simulink library "body_chassis_vert"  (R2018b)
settings: Solver=ode45  StartTime=0.0  StopTime=10.0  RelTol=1e-3  EnableMultiTasking=on
undefined symbols (not defined in the file): DiscIntNeverNeededParam, par_VEH, phi0, psip0, stepsize, v0
libraries: $bdroot x4
(part 2 of 2)

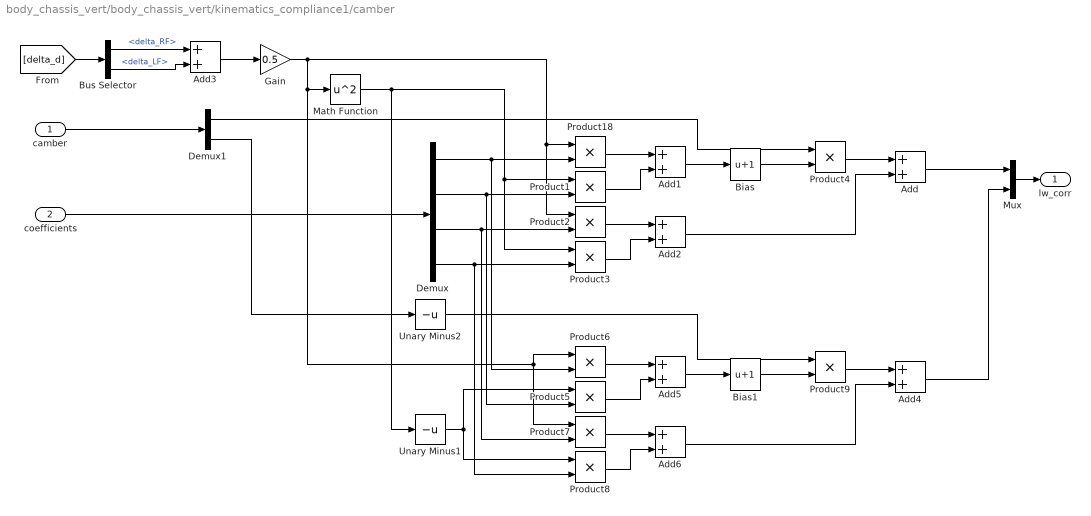
== system body_chassis_vert/body_chassis_vert/kinematics_compliance1/camber ==
  "camber " : Inport
  coefficients : Inport  Port=2
  Add{,1..6} (7 alike) : Sum
  Bias : Bias  Bias=1
  Bias1 : Bias  Bias=1
  Bus Selector : BusSelector  OutputSignals=delta_RF,delta_LF
  Demux : Demux
  Demux1 : Demux  Outputs=2
  Gain : Gain  Gain=0.5
  Math Function : Math  Operator=square  SaturateOnIntegerOverflow=on
  Mux : Mux  Inputs=2
  Product{1..9,18} (10 alike) : Product  RndMeth=Zero
  Unary Minus1 : UnaryMinus
  Unary Minus2 : UnaryMinus
  lw_corr : Outport
  wires:
  Unary Minus2/1 -> Product9/1
  Add3/1 -> Gain/1
  Bus Selector/2 -> Add3/2  "<delta_LF>"
  Bus Selector/1 -> Add3/1  "<delta_RF>"
  [delta_d] -> Bus Selector/1
  "camber "/1 -> Demux1/1
  Add/1 -> Mux/1
  coefficients/1 -> Demux/1
  Demux/1 -> Product6/2, Product18/2
  Demux/2 -> Product5/2, Product1/2
  Math Function/1 -> Unary Minus1/1, Product3/1, Product1/1
  Demux/3 -> Product7/2, Product2/2
  Demux/4 -> Product8/2, Product3/2
  Product18/1 -> Add1/1
  Product1/1 -> Add1/2
  Add1/1 -> Bias/1
  Product2/1 -> Add2/1
  Product3/1 -> Add2/2
  Add2/1 -> Add/2
  Bias/1 -> Product4/2
  Product4/1 -> Add/1
  Demux1/1 -> Product4/1
  Add4/1 -> Mux/2
  Product5/1 -> Add5/2
  Add5/1 -> Bias1/1
  Product7/1 -> Add6/1
  Product8/1 -> Add6/2
  Add6/1 -> Add4/2
  Bias1/1 -> Product9/2
  Product9/1 -> Add4/1
  Gain/1 -> Math Function/1, Product6/1, Product7/1, Product2/1, Product18/1
  Unary Minus1/1 -> Product5/1, Product8/1
  Product6/1 -> Add5/1
  Demux1/2 -> Unary Minus2/1
  Mux/1 -> lw_corr/1

== system body_chassis_vert/body_chassis_vert/kinematics_compliance1/toe ==
  "toe " : Inport
  coefficients : Inport  Port=2
  Add{,1..6} (7 alike) : Sum
  Bias : Bias  Bias=1
  Bias1 : Bias  Bias=1
  Bus Selector : BusSelector  OutputSignals=delta_RF,delta_LF
  Demux : Demux
  Demux1 : Demux  Outputs=2
  Gain : Gain  Gain=0.5
  Math Function : Math  Operator=square  SaturateOnIntegerOverflow=on
  Mux : Mux  Inputs=2
  Product{1..9,18} (10 alike) : Product  RndMeth=Zero
  Unary Minus : UnaryMinus
  Unary Minus2 : UnaryMinus
  lw_corr : Outport
  wires:
  Unary Minus2/1 -> Product9/1
  Mux/1 -> lw_corr/1
  Demux1/2 -> Unary Minus2/1
  Product6/1 -> Add5/1
  Math Function/1 -> Product1/1, Product3/1, Product5/1, Product8/1
  Unary Minus/1 -> Product7/1, Product6/1
  Product9/1 -> Add4/1
  Bias1/1 -> Product9/2
  Add6/1 -> Add4/2
  Product8/1 -> Add6/2
  Product7/1 -> Add6/1
  Add5/1 -> Bias1/1
  Product5/1 -> Add5/2
  Add4/1 -> Mux/2
  Demux1/1 -> Product4/1
  Product4/1 -> Add/1
  Bias/1 -> Product4/2
  Add2/1 -> Add/2
  Product3/1 -> Add2/2
  Product2/1 -> Add2/1
  Add1/1 -> Bias/1
  Product1/1 -> Add1/2
  Product18/1 -> Add1/1
  Demux/4 -> Product3/2, Product8/2
  Demux/3 -> Product2/2, Product7/2
  Demux/2 -> Product1/2, Product5/2
  Gain/1 -> Product18/1, Product2/1, Math Function/1, Unary Minus/1
  Demux/1 -> Product18/2, Product6/2
  coefficients/1 -> Demux/1
  Add/1 -> Mux/1
  "toe "/1 -> Demux1/1
  [delta_d] -> Bus Selector/1
  Bus Selector/1 -> Add3/1  "<delta_RF>"
  Bus Selector/2 -> Add3/2  "<delta_LF>"
  Add3/1 -> Gain/1

== system body_chassis_vert/body_chassis_vert/roll/phi ==
  phi : Inport
  LF : Inport  Port=2
  RF : Inport  Port=3
  RR : Inport  Port=4
  LR : Inport  Port=5
  Product{5..8} (4 alike) : Product  RndMeth=Zero
  Trigonometric Function : Trigonometry
  Unary Minus1 : UnaryMinus
  RF_out : Outport
  LF_out : Outport  Port=2
  RR_out : Outport  Port=3
  LR_out : Outport  Port=4
  wires:
  Product8/1 -> LR_out/1  "z_roll_LR"
  Product7/1 -> RR_out/1  "z_roll_RR"
  Product6/1 -> LF_out/1  "z_roll_LF"
  Product5/1 -> RF_out/1  "z_roll_RF"
  LR/1 -> Product8/2
  RR/1 -> Product7/2
  LF/1 -> Product6/2
  RF/1 -> Product5/2
  phi/1 -> Trigonometric Function/1
  Trigonometric Function/1 -> Product8/1, Product6/1, Unary Minus1/1
  Unary Minus1/1 -> Product5/1, Product7/1

== system body_chassis_vert/body_chassis_vert/suspension/arb ==
  note: Fz_arb_RF is refered to wheel
  z_roll : Inport
  z_wheel_vert : Inport  Port=2
  Bus Creator : BusCreator  Inputs=4
  Front : Subsystem
  Front1 : Subsystem
  F_arb : Outport
  wires:
  [carbR] -> Front1/3(carb)
  Front/2(Fz_arb_L) -> Bus Creator/2  "Fz_arb_LF"
  z_wheel_vert/1 -> Front1/2(z_wheel_vert), Front/2(z_wheel_vert)
  z_roll/1 -> Front1/1(z_roll), Front/1(z_roll)
  Front1/2(Fz_arb_L) -> Bus Creator/4  "Fz_arb_LR"
  Front1/1(Fz_arb_R) -> Bus Creator/3  "Fz_arb_RR"
  Front/1(Fz_arb_R) -> Bus Creator/1  "Fz_arb_RF"
  Bus Creator/1 -> F_arb/1
  [carbF] -> Front/3(carb)

== system body_chassis_vert/body_chassis_vert/suspension/damper ==
  note: Fz_damper is refered to wheel
  z_roll : Inport
  z_pitch : Inport  Port=2
  z_body_vert : Inport  Port=3
  z_wheel_vert : Inport  Port=4
  Bus Creator : BusCreator  Inputs=4
  Bus Creator1 : BusCreator  Inputs=4
  Bus Selector : BusSelector  OutputSignals=z_roll_RF.z_roll_RFp,z_roll_LF.z_roll_LFp,z_roll_RR.z_roll_RRp,z_roll_LR.z_roll_LRp
  Bus Selector1 : BusSelector  OutputSignals=z_pitch_RF.z_pitch_RFp,z_pitch_LF.z_pitch_LFp,z_pitch_RR.z_pitch_RRp,z_pitch_LR.z_pitch_LRp
  Bus Selector2 : BusSelector  OutputSignals=z_vertp
  Bus Selector3 : BusSelector  OutputSignals=zwheel_RF.zwheelp,zwheel_LF.zwheelp,zwheel_RR.zwheelp,zwheel_LR.zwheelp
  LF : Subsystem
  LR : Subsystem
  RF : Subsystem
  RR : Subsystem
  F_damper : Outport
  P_damper : Outport  Port=2
  wires:
  Bus Selector3/3 -> RR/4(z_wheel_vertp)  "<zwheelp>"
  Bus Selector3/2 -> LF/4(z_wheel_vertp)  "<zwheelp>"
  Bus Selector3/1 -> RF/4(z_wheel_vertp)  "<zwheelp>"
  Bus Selector/4 -> LR/1(z_rollp)  "<z_roll_LRp>"
  Bus Selector/3 -> RR/1(z_rollp)  "<z_roll_RRp>"
  Bus Selector/2 -> LF/1(z_rollp)  "<z_roll_LFp>"
  Bus Selector/1 -> RF/1(z_rollp)  "<z_roll_RFp>"
  Bus Selector1/1 -> RF/2(z_pitchp)  "<z_pitch_RFp>"
  Bus Selector1/2 -> LF/2(z_pitchp)  "<z_pitch_LFp>"
  Bus Selector1/3 -> RR/2(z_pitchp)  "<z_pitch_RRp>"
  Bus Selector1/4 -> LR/2(z_pitchp)  "<z_pitch_LRp>"
  Bus Selector3/4 -> LR/4(z_wheel_vertp)  "<zwheelp>"
  Bus Selector2/1 -> LR/3(z_vertp), RR/3(z_vertp), LF/3(z_vertp), RF/3(z_vertp)  "<z_vertp>"
  z_body_vert/1 -> Bus Selector2/1
  RF/1(Fz_damper) -> Bus Creator/1  "Fz_damper_RF"
  LF/1(Fz_damper) -> Bus Creator/2  "Fz_damper_LF"
  RR/1(Fz_damper) -> Bus Creator/3  "Fz_damper_RR"
  LR/1(Fz_damper) -> Bus Creator/4  "Fz_damper_LR"
  z_roll/1 -> Bus Selector/1
  z_pitch/1 -> Bus Selector1/1
  Bus Creator/1 -> F_damper/1
  z_wheel_vert/1 -> Bus Selector3/1
  Bus Creator1/1 -> P_damper/1
  RF/2(P_damper) -> Bus Creator1/1  "P_damper_RF"
  LF/2(P_damper) -> Bus Creator1/2  "P_damper_LF"
  RR/2(P_damper) -> Bus Creator1/3  "P_damper_RR"
  LR/2(P_damper) -> Bus Creator1/4  "P_damper_LR"

== system body_chassis_vert/body_chassis_vert/suspension/spring ==
  note: Fz_spring is refered to wheel
  z_roll : Inport
  z_pitch : Inport  Port=2
  z_vert : Inport  Port=3
  z_wheel_vert : Inport  Port=4
  Bus Creator : BusCreator  Inputs=4
  Bus Creator1 : BusCreator  Inputs=4
  Bus Selector : BusSelector  OutputSignals=z_roll_RF.z_roll_RF,z_roll_LF.z_roll_LF,z_roll_RR.z_roll_RR,z_roll_LR.z_roll_LR
  Bus Selector1 : BusSelector  OutputSignals=z_pitch_RF.z_pitch_RF,z_pitch_LF.z_pitch_LF,z_pitch_RR.z_pitch_RR,z_pitch_LR.z_pitch_LR
  Bus Selector2 : BusSelector  OutputSignals=z_vert
  Bus Selector3 : BusSelector  OutputSignals=zwheel_RF.zwheel,zwheel_LF.zwheel,zwheel_RR.zwheel,zwheel_LR.zwheel
  LF : $bdroot/body_chassis_vert/suspension/spring/RF  SystemSampleTime=-1
  LR : $bdroot/body_chassis_vert/suspension/spring/RR  SystemSampleTime=-1
  RF : Subsystem
  RR : Subsystem
  Fz_spring : Outport
  z_wheel : Outport  Port=2
  wires:
  z_pitch/1 -> Bus Selector1/1
  LR/2 -> Bus Creator1/4  "z_wheel_LR"
  RR/2(z_wheel) -> Bus Creator1/3  "z_wheel_RR"
  LF/2 -> Bus Creator1/2  "z_wheel_LF"
  RF/2(z_wheel) -> Bus Creator1/1  "z_wheel_RF"
  Bus Creator1/1 -> z_wheel/1
  Bus Selector2/1 -> RF/3(z_vert), LF/3, LR/2, RR/3(z_vert)  "<z_vert>"
  Bus Selector3/4 -> LR/4  "<zwheel>"
  Bus Selector3/3 -> RR/4(z_wheel_vert)  "<zwheel>"
  z_wheel_vert/1 -> Bus Selector3/1
  Bus Selector3/1 -> RF/4(z_wheel_vert)  "<zwheel>"
  z_vert/1 -> Bus Selector2/1
  Bus Creator/1 -> Fz_spring/1
  Bus Selector1/4 -> LR/3  "<z_pitch_LR>"
  Bus Selector1/3 -> RR/2(z_pitch)  "<z_pitch_RR>"
  Bus Selector1/2 -> LF/2  "<z_pitch_LF>"
  Bus Selector1/1 -> RF/2(z_pitch)  "<z_pitch_RF>"
  Bus Selector/4 -> LR/1  "<z_roll_LR>"
  Bus Selector/3 -> RR/1(z_roll)  "<z_roll_RR>"
  z_roll/1 -> Bus Selector/1
  Bus Selector/2 -> LF/1  "<z_roll_LF>"
  Bus Selector/1 -> RF/1(z_roll)  "<z_roll_RF>"
  LR/1 -> Bus Creator/4  "Fz_spring_LR"
  RR/1(Fz_spring) -> Bus Creator/3  "Fz_spring_RR"
  LF/1 -> Bus Creator/2  "Fz_spring_LF"
  RF/1(Fz_spring) -> Bus Creator/1  "Fz_spring_RF"
  Bus Selector3/2 -> LF/4  "<zwheel>"

== system body_chassis_vert/body_chassis_vert/horizontal/betap/Blending ==
  betapin : Inport
  absVx : Inport  Port=2
  Bias : Bias  Bias=1
  Bias1 : Bias  Bias=-2*pi
  Gain : Gain  Gain=2*pi*0.5
  Gain1 : Gain  Gain=0.5
  Product : Product  RndMeth=Zero
  Trigonometric Function : Trigonometry  Operator=tanh
  betapout : Outport
  wires:
  Gain1/1 -> Product/1
  Bias/1 -> Gain1/1
  Trigonometric Function/1 -> Bias/1
  Bias1/1 -> Trigonometric Function/1
  Gain/1 -> Bias1/1
  absVx/1 -> Gain/1
  Product/1 -> betapout/1
  betapin/1 -> Product/2

== system body_chassis_vert/body_chassis_vert/suspension/arb/Front ==
  z_roll : Inport
  z_wheel_vert : Inport  Port=2
  carb : Inport  Port=3
  Add : Sum  Inputs=+--+
  Bus Selector : BusSelector  OutputSignals=z_roll_RF.z_roll_RF,z_roll_LF.z_roll_LF
  Bus Selector1 : BusSelector  OutputSignals=zwheel_RF.zwheel,zwheel_LF.zwheel
  Divide : Product  Inputs=*/
  Gain : Gain  Gain=0.5
  Product : Product  RndMeth=Zero
  Product1 : Product  Inputs=3  RndMeth=Zero
  Unary Minus1 : UnaryMinus
  Fz_arb_R : Outport
  Fz_arb_L : Outport  Port=2
  wires:
  Gain/1 -> Product/2
  Product1/1 -> Gain/1
  carb/1 -> Product1/1
  Divide/1 -> Product1/2, Product1/3
  [sF] -> Divide/2
  [sarbF] -> Divide/1
  Bus Selector1/2 -> Add/4  "<zwheel>"
  Bus Selector1/1 -> Add/3  "<zwheel>"
  Bus Selector/2 -> Add/2  "<z_roll_LF>"
  Bus Selector/1 -> Add/1  "<z_roll_RF>"
  z_wheel_vert/1 -> Bus Selector1/1
  z_roll/1 -> Bus Selector/1
  Add/1 -> Product/1
  Unary Minus1/1 -> Fz_arb_R/1
  Product/1 -> Fz_arb_L/1, Unary Minus1/1

== system body_chassis_vert/body_chassis_vert/suspension/arb/Front1 ==
  z_roll : Inport
  z_wheel_vert : Inport  Port=2
  carb : Inport  Port=3
  Add : Sum  Inputs=+--+
  Bus Selector : BusSelector  OutputSignals=z_roll_RR.z_roll_RR,z_roll_LR.z_roll_LR
  Bus Selector1 : BusSelector  OutputSignals=zwheel_RR.zwheel,zwheel_LR.zwheel
  Divide : Product  Inputs=*/
  Gain : Gain  Gain=0.5
  Product : Product  RndMeth=Zero
  Product1 : Product  Inputs=3  RndMeth=Zero
  Unary Minus1 : UnaryMinus
  Fz_arb_R : Outport
  Fz_arb_L : Outport  Port=2
  wires:
  Product/1 -> Unary Minus1/1, Fz_arb_L/1
  Unary Minus1/1 -> Fz_arb_R/1
  Add/1 -> Product/1
  z_roll/1 -> Bus Selector/1
  z_wheel_vert/1 -> Bus Selector1/1
  Bus Selector/1 -> Add/1  "<z_roll_RR>"
  Bus Selector/2 -> Add/2  "<z_roll_LR>"
  Bus Selector1/1 -> Add/3  "<zwheel>"
  Bus Selector1/2 -> Add/4  "<zwheel>"
  [sarbR] -> Divide/1
  [sR] -> Divide/2
  Divide/1 -> Product1/3, Product1/2
  carb/1 -> Product1/1
  Product1/1 -> Gain/1
  Gain/1 -> Product/2

== system body_chassis_vert/body_chassis_vert/suspension/damper/LF ==
  z_rollp : Inport
  z_pitchp : Inport  Port=2
  z_vertp : Inport  Port=3
  z_wheel_vertp : Inport  Port=4
  Add : Sum  Inputs=+++-
  Divide : Product  Inputs=*/
  Product1 : Product  RndMeth=Zero
  Product2 : Product  RndMeth=Zero
  Product3 : Product  RndMeth=Zero
  Switch : Switch
  compression : Polyval  Coefs=par_VEH.ddF_comp
  rebound : Polyval  Coefs=par_VEH.ddF_reb
  Fz_damper : Outport
  P_damper : Outport  Port=2
  wires:
  Add/1 -> Product3/1
  rebound/1 -> Switch/1
  compression/1 -> Switch/3
  Product2/1 -> Fz_damper/1
  Divide/1 -> Product3/2, Product2/2
  [sF] -> Divide/2
  [sdF] -> Divide/1
  z_vertp/1 -> Add/3
  z_rollp/1 -> Add/1
  z_pitchp/1 -> Add/2
  z_wheel_vertp/1 -> Add/4
  Switch/1 -> Product1/1, Product2/1
  Product3/1 -> Switch/2, rebound/1, compression/1, Product1/2
  Product1/1 -> P_damper/1

== system body_chassis_vert/body_chassis_vert/suspension/damper/LR ==
  z_rollp : Inport
  z_pitchp : Inport  Port=2
  z_vertp : Inport  Port=3
  z_wheel_vertp : Inport  Port=4
  Add : Sum  Inputs=+++-
  Divide : Product  Inputs=*/
  Product1 : Product  RndMeth=Zero
  Product2 : Product  RndMeth=Zero
  Product3 : Product  RndMeth=Zero
  Switch : Switch
  compression : Polyval  Coefs=par_VEH.ddR_comp
  rebound : Polyval  Coefs=par_VEH.ddR_reb
  Fz_damper : Outport
  P_damper : Outport  Port=2
  wires:
  Add/1 -> Product3/1
  rebound/1 -> Switch/1
  compression/1 -> Switch/3
  Product2/1 -> Fz_damper/1
  Divide/1 -> Product2/2, Product3/2
  [sR] -> Divide/2
  [sdR] -> Divide/1
  z_vertp/1 -> Add/3
  z_rollp/1 -> Add/1
  z_pitchp/1 -> Add/2
  z_wheel_vertp/1 -> Add/4
  Switch/1 -> Product1/1, Product2/1
  Product3/1 -> Product1/2, compression/1, Switch/2, rebound/1
  Product1/1 -> P_damper/1

== system body_chassis_vert/body_chassis_vert/suspension/damper/RF ==
  z_rollp : Inport
  z_pitchp : Inport  Port=2
  z_vertp : Inport  Port=3
  z_wheel_vertp : Inport  Port=4
  Add : Sum  Inputs=+++-
  Divide : Product  Inputs=*/
  Product1 : Product  RndMeth=Zero
  Product2 : Product  RndMeth=Zero
  Product3 : Product  RndMeth=Zero
  Switch : Switch
  compression : Polyval  Coefs=par_VEH.ddF_comp
  rebound : Polyval  Coefs=par_VEH.ddF_reb
  Fz_damper : Outport
  P_damper : Outport  Port=2
  wires:
  Product3/1 -> rebound/1, Switch/2, compression/1, Product1/2
  Add/1 -> Product3/1
  Switch/1 -> Product1/1, Product2/1
  rebound/1 -> Switch/1
  compression/1 -> Switch/3
  Product2/1 -> Fz_damper/1
  Divide/1 -> Product3/2, Product2/2
  [sF] -> Divide/2
  [sdF] -> Divide/1
  z_vertp/1 -> Add/3
  z_rollp/1 -> Add/1
  z_pitchp/1 -> Add/2
  z_wheel_vertp/1 -> Add/4
  Product1/1 -> P_damper/1

== system body_chassis_vert/body_chassis_vert/suspension/damper/RR ==
  z_rollp : Inport
  z_pitchp : Inport  Port=2
  z_vertp : Inport  Port=3
  z_wheel_vertp : Inport  Port=4
  Add : Sum  Inputs=+++-
  Divide : Product  Inputs=*/
  Product1 : Product  RndMeth=Zero
  Product2 : Product  RndMeth=Zero
  Product3 : Product  RndMeth=Zero
  Switch : Switch
  compression : Polyval  Coefs=par_VEH.ddR_comp
  rebound : Polyval  Coefs=par_VEH.ddR_reb
  Fz_damper : Outport
  P_damper : Outport  Port=2
  wires:
  Add/1 -> Product3/1
  rebound/1 -> Switch/1
  compression/1 -> Switch/3
  Product2/1 -> Fz_damper/1
  Divide/1 -> Product2/2, Product3/2
  [sR] -> Divide/2
  [sdR] -> Divide/1
  z_vertp/1 -> Add/3
  z_rollp/1 -> Add/1
  z_pitchp/1 -> Add/2
  z_wheel_vertp/1 -> Add/4
  Switch/1 -> Product1/1, Product2/1
  Product3/1 -> Switch/2, rebound/1, Product1/2, compression/1
  Product1/1 -> P_damper/1

== system body_chassis_vert/body_chassis_vert/suspension/spring/RF ==
  z_roll : Inport
  z_pitch : Inport  Port=2
  z_vert : Inport  Port=3
  z_wheel_vert : Inport  Port=4
  Add : Sum  Inputs=---+
  Divide : Product  Inputs=*/
  Product : Product
  Product1 : Product
  csRF : Lookup_n-D  NumberOfTableDimensions=1  BreakpointsForDimension1=par_VEH.cF_front(:,1)  Table=par_VEH.cF_front(:,2)  InternalRulePriority=Speed  RndMeth=Simplest  InputSameDT=on
  Fz_spring : Outport
  z_wheel : Outport  Port=2
  wires:
  csRF/1 -> Product1/1
  Divide/1 -> Product/2, Product1/2
  Product/1 -> csRF/1
  [sF] -> Divide/2
  [ssF] -> Divide/1
  z_wheel_vert/1 -> Add/4
  z_vert/1 -> Add/3
  z_pitch/1 -> Add/2
  z_roll/1 -> Add/1
  Add/1 -> z_wheel/1, Product/1
  Product1/1 -> Fz_spring/1

== system body_chassis_vert/body_chassis_vert/suspension/spring/RR ==
  z_roll : Inport
  z_pitch : Inport  Port=2
  z_vert : Inport  Port=3
  z_wheel_vert : Inport  Port=4
  Add : Sum  Inputs=---+
  Divide : Product  Inputs=*/
  Product : Product
  Product1 : Product
  csRF : Lookup_n-D  NumberOfTableDimensions=1  BreakpointsForDimension1=par_VEH.cF_rear(:,1)  Table=par_VEH.cF_rear(:,2)  InternalRulePriority=Speed  RndMeth=Simplest  InputSameDT=on
  Fz_spring : Outport
  z_wheel : Outport  Port=2
  wires:
  Product1/1 -> Fz_spring/1
  Product/1 -> csRF/1
  Divide/1 -> Product/2, Product1/2
  [sR] -> Divide/2
  [ssR] -> Divide/1
  z_wheel_vert/1 -> Add/4
  z_vert/1 -> Add/3
  z_pitch/1 -> Add/2
  z_roll/1 -> Add/1
  Add/1 -> z_wheel/1, Product/1
  csRF/1 -> Product1/1
